simulink model "Allocation_Complex"  (R2015a)
settings: Solver=ode45  StartTime=0.0  StopTime=10.0  RelTol=1e-3
undefined symbols (not defined in the file or in its folder): magnitude
libraries: simulink x16, aerolibutil x10, simulink_extras x6
settings Model: Creator=Nick  LastModifiedBy=Nick

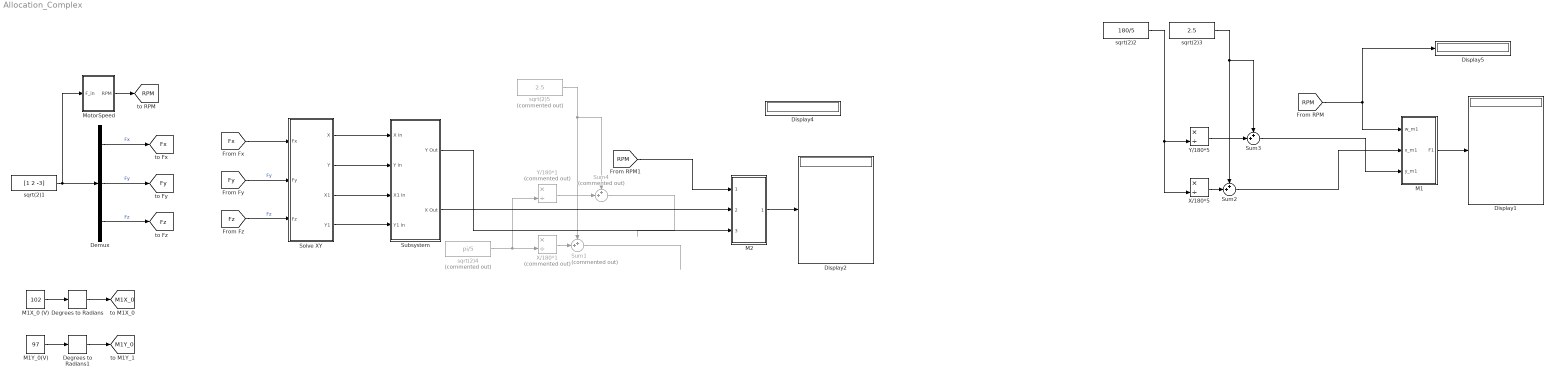
== system Allocation_Complex ==
  Degrees to Radians : simulink_extras/Transformations/Degrees to Radians
  Degrees to Radians1 : simulink_extras/Transformations/Degrees to Radians
  Demux : Demux  Outputs=3
  Display{1..2,4..5} (4 alike) : Display
      settings: Decimation=4
  M1 : Subsystem
  M1X_0 (V) : Constant  Value=102
  M1Y_0(V) : Constant  Value=97
  M2 : Subsystem
  MotorSpeed : Subsystem
  Solve XY : Subsystem
  Subsystem : Subsystem
  Sum1 : Sum  Commented=on  Inputs=++|
  Sum2 : Sum  Inputs=++|
  Sum3 : Sum  Inputs=++|
  Sum4 : Sum  Commented=on  Inputs=++|
  X/180*1 : Product  Commented=on  Inputs=*/
  X/180*5 : Product  Inputs=*/
  Y/180*1 : Product  Commented=on  Inputs=*/
  Y/180*5 : Product  Inputs=*/
  sqrt(2)1 : Constant  Value=[1 2 -3]
  sqrt(2)2 : Constant  Value=180/5
  sqrt(2)3 : Constant  Value=2.5
  sqrt(2)4 : Constant  Commented=on  Value=pi/5
  sqrt(2)5 : Constant  Commented=on  Value=2.5
  tag scope: Fx=global, Fy=global, Fz=global, M1X_0=global, M1Y_0=global, RPM=global
  wires:
  [RPM] -> M1/1(w_m1), Display5/1
  sqrt(2)1/1 -> Demux/1, MotorSpeed/1(F_in)
  sqrt(2)2/1 -> Y/180*5/2, X/180*5/2
  X/180*5/1 -> Sum2/2
  Y/180*5/1 -> Sum3/2
  sqrt(2)3/1 -> Sum3/1, Sum2/1
  M1/1(F1) -> Display1/1
  Sum3/1 -> M1/3(y_m1)
  Sum2/1 -> M1/2(x_m1)
  Demux/1 -> [Fx]  "Fx"
  Demux/2 -> [Fy]  "Fy"
  Demux/3 -> [Fz]  "Fz"
  MotorSpeed/1(RPM) -> [RPM]
  [Fz] -> Solve XY/3(Fz)  "Fz"
  [Fx] -> Solve XY/1(Fx)
  [Fy] -> Solve XY/2(Fy)  "Fy"
  Solve XY/4(Y1) -> Subsystem/4(Y1 in)
  Solve XY/3(X1) -> Subsystem/3(X1 in)
  Solve XY/2(Y) -> Subsystem/2(Y in)
  Solve XY/1(X) -> Subsystem/1(X in)
  M1X_0 (V)/1 -> Degrees to Radians/1
  Degrees to Radians/1 -> [M1X_0]
  M1Y_0(V)/1 -> Degrees to Radians1/1
  Degrees to Radians1/1 -> [M1Y_0]
  [RPM] -> M2/1(w_m1)
  sqrt(2)4/1 -> Y/180*1/2, X/180*1/2
  X/180*1/1 -> Sum1/2
  Y/180*1/1 -> Sum4/2
  sqrt(2)5/1 -> Sum4/1, Sum1/1
  M2/1(Fz_m1) -> Display2/1
  Sum1/1 -> ?
  Sum4/1 -> ?
  Subsystem/1(Y Out) -> M2/3(y_m1)
  Subsystem/2(X Out) -> M2/2(x_m1)

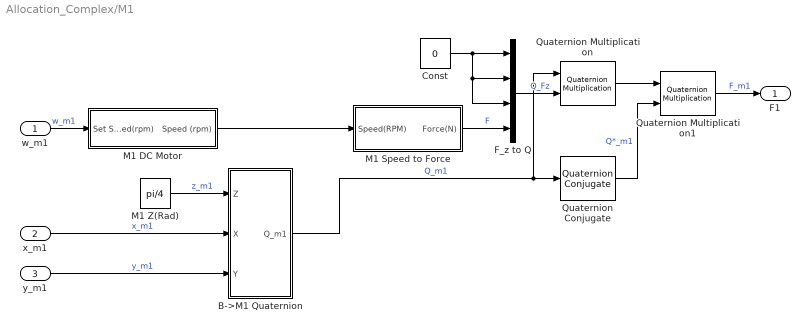
== system Allocation_Complex/M1 ==
  w_m1 : Inport
  x_m1 : Inport  Port=2
  y_m1 : Inport  Port=3
  B->M1 Quaternion : Subsystem
  Const : Constant  Value=0
  F_z to Q : Concatenate  NumInputs=4
  M1 DC Motor : Subsystem
  M1 Speed to Force : Subsystem
  M1 Z(Rad) : Constant  Value=pi/4
  Quaternion Conjugate : aerolibutil/Quaternion Conjugate
  Quaternion Multiplication : aerolibutil/Quaternion Multiplication
  Quaternion Multiplication1 : aerolibutil/Quaternion Multiplication
  F1 : Outport
  wires:
  Quaternion Multiplication/1 -> Quaternion Multiplication1/1
  Const/1 -> F_z to Q/1, F_z to Q/3, F_z to Q/2
  M1 DC Motor/1(Speed (rpm)) -> M1 Speed to Force/1(Speed(RPM))
  B->M1 Quaternion/1(Q_m1) -> Quaternion Conjugate/1, Quaternion Multiplication/1  "Q_m1"
  w_m1/1 -> M1 DC Motor/1(Set Speed(rpm))  "w_m1"
  F_z to Q/1 -> Quaternion Multiplication/2  "Q_Fz"
  M1 Z(Rad)/1 -> B->M1 Quaternion/1("Z ")  "z_m1"
  M1 Speed to Force/1(Force(N)) -> F_z to Q/4  "F"
  y_m1/1 -> B->M1 Quaternion/3(Y)  "y_m1"
  Quaternion Conjugate/1 -> Quaternion Multiplication1/2  "Q*_m1"
  Quaternion Multiplication1/1 -> F1/1  "F_m1"
  x_m1/1 -> B->M1 Quaternion/2(X)  "x_m1"

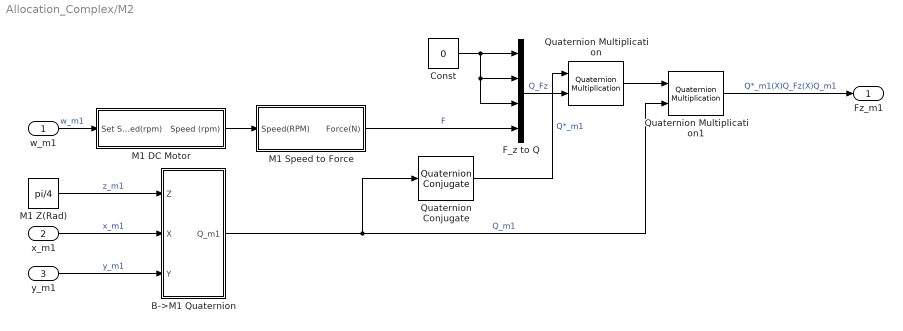
== system Allocation_Complex/M2 ==
  w_m1 : Inport
  x_m1 : Inport  Port=2
  y_m1 : Inport  Port=3
  B->M1 Quaternion : Subsystem
  Const : Constant  Value=0
  F_z to Q : Concatenate  NumInputs=4
  M1 DC Motor : Subsystem
  M1 Speed to Force : Subsystem
  M1 Z(Rad) : Constant  Value=pi/4
  Quaternion Conjugate : aerolibutil/Quaternion Conjugate
  Quaternion Multiplication : aerolibutil/Quaternion Multiplication
  Quaternion Multiplication1 : aerolibutil/Quaternion Multiplication
  Fz_m1 : Outport
  wires:
  Quaternion Multiplication/1 -> Quaternion Multiplication1/1
  Const/1 -> F_z to Q/1, F_z to Q/3, F_z to Q/2
  M1 DC Motor/1(Speed (rpm)) -> M1 Speed to Force/1(Speed(RPM))
  B->M1 Quaternion/1(Q_m1) -> Quaternion Multiplication1/2, Quaternion Conjugate/1  "Q_m1"
  w_m1/1 -> M1 DC Motor/1(Set Speed(rpm))  "w_m1"
  F_z to Q/1 -> Quaternion Multiplication/2  "Q_Fz"
  M1 Z(Rad)/1 -> B->M1 Quaternion/1("Z ")  "z_m1"
  M1 Speed to Force/1(Force(N)) -> F_z to Q/4  "F"
  y_m1/1 -> B->M1 Quaternion/3(Y)  "y_m1"
  Quaternion Multiplication1/1 -> Fz_m1/1  "Q*_m1(X)Q_Fz(X)Q_m1"
  x_m1/1 -> B->M1 Quaternion/2(X)  "x_m1"
  Quaternion Conjugate/1 -> Quaternion Multiplication/1  "Q*_m1"

== system Allocation_Complex/MotorSpeed ==
  F_in : Inport
  Divide : Product  Inputs=*/
  Force Coefficient CT : Constant  Value=0.000243
  Mins : Constant  Value=60
  Product : Product
  w^2 : Sqrt  SaturateOnIntegerOverflow=on
  |F| : Sqrt  SaturateOnIntegerOverflow=on
  |F|^2 : DotProduct  InputSameDT=on  OutDataTypeStr=Inherit: Inherit via internal rule
  RPM : Outport
  wires:
  w^2/1 -> Product/2
  Product/1 -> RPM/1  "RPM"
  Mins/1 -> Product/1
  Divide/1 -> w^2/1
  Force Coefficient CT/1 -> Divide/2
  F_in/1 -> |F|^2/2, |F|^2/1
  |F|^2/1 -> |F|/1
  |F|/1 -> Divide/1

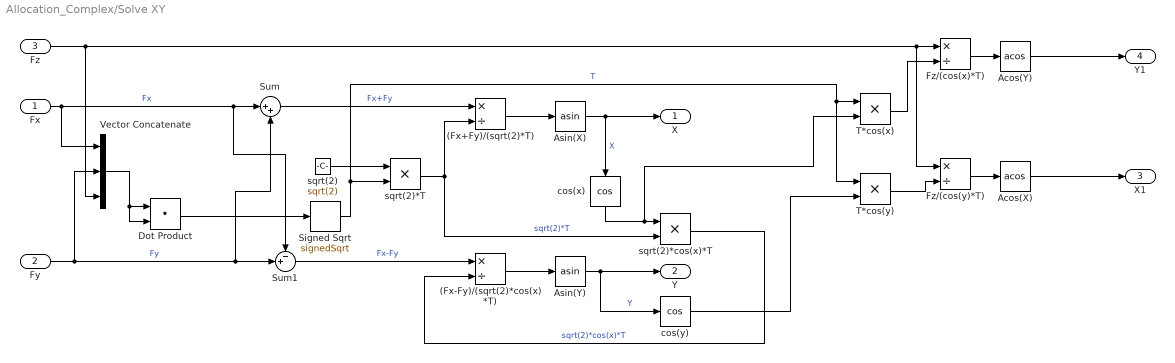
== system Allocation_Complex/Solve XY ==
  Fx : Inport
  Fy : Inport  Port=2
  Fz : Inport  Port=3
  (Fx+Fy)/(sqrt(2)*T) : Product  Inputs=*/
  (Fx-Fy)/(sqrt(2)*cos(x)*T) : Product  Inputs=*/
  Acos(X) : Trigonometry  Operator=acos
  Acos(Y) : Trigonometry  Operator=acos
  Asin(X) : Trigonometry  Operator=asin
  Asin(Y) : Trigonometry  Operator=asin
  Dot Product : DotProduct  InputSameDT=on  OutDataTypeStr=Inherit: Inherit via internal rule
  Fz/(cos(x)*T) : Product  Inputs=*/
  Fz/(cos(y)*T) : Product  Inputs=*/
  Signed Sqrt : Sqrt  Operator=signedSqrt  SaturateOnIntegerOverflow=on
  Sum : Sum  Inputs=|++
  Sum1 : Sum  Inputs=-+|
  T*cos(x) : Product
  T*cos(y) : Product
  Vector Concatenate : Concatenate  NumInputs=3
  cos(x) : Trigonometry  Operator=cos
  cos(y) : Trigonometry  Operator=cos
  sqrt(2) : Constant  Value=sqrt(2)
  sqrt(2)*T : Product
  sqrt(2)*cos(x)*T : Product
  X : Outport
  Y : Outport  Port=2
  X1 : Outport  Port=3
  Y1 : Outport  Port=4
  wires:
  Fy/1 -> Vector Concatenate/2, Sum/2, Sum1/2  "Fy"
  Sum/1 -> (Fx+Fy)/(sqrt(2)*T)/1  "Fx+Fy"
  sqrt(2)/1 -> sqrt(2)*T/1
  T*cos(x)/1 -> Fz/(cos(x)*T)/2
  cos(x)/1 -> sqrt(2)*cos(x)*T/1, T*cos(x)/2
  sqrt(2)*T/1 -> (Fx+Fy)/(sqrt(2)*T)/2, sqrt(2)*cos(x)*T/2  "sqrt(2)*T"
  Fz/(cos(y)*T)/1 -> Acos(X)/1
  (Fx+Fy)/(sqrt(2)*T)/1 -> Asin(X)/1
  cos(y)/1 -> T*cos(y)/2
  sqrt(2)*cos(x)*T/1 -> (Fx-Fy)/(sqrt(2)*cos(x)*T)/2  "sqrt(2)*cos(x)*T"
  (Fx-Fy)/(sqrt(2)*cos(x)*T)/1 -> Asin(Y)/1
  Sum1/1 -> (Fx-Fy)/(sqrt(2)*cos(x)*T)/1  "Fx-Fy"
  Acos(Y)/1 -> Y1/1
  Asin(Y)/1 -> Y/1, cos(y)/1  "Y"
  Fz/(cos(x)*T)/1 -> Acos(Y)/1
  T*cos(y)/1 -> Fz/(cos(y)*T)/2
  Acos(X)/1 -> X1/1
  Asin(X)/1 -> X/1, cos(x)/1  "X"
  Fz/1 -> Vector Concatenate/3, Fz/(cos(y)*T)/1, Fz/(cos(x)*T)/1
  Signed Sqrt/1 -> T*cos(x)/1, T*cos(y)/1, sqrt(2)*T/2  "T"
  Fx/1 -> Sum1/1, Sum/1, Vector Concatenate/1  "Fx"
  Vector Concatenate/1 -> Dot Product/2, Dot Product/1
  Dot Product/1 -> Signed Sqrt/1

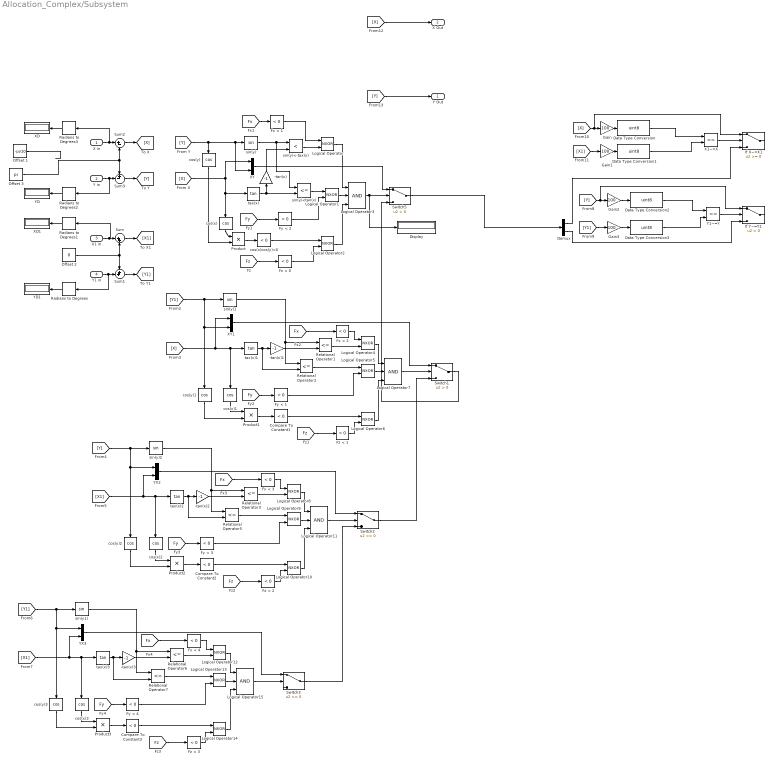
== system Allocation_Complex/Subsystem ==
  X in : Inport
  Y in : Inport  Port=2
  X1 in : Inport  Port=3
  Y1 in : Inport  Port=4
  -tan(x){,1..3} (4 alike) : Gain  Gain=-1
  Compare To Constant1 : simulink/Logic and Bit Operations/Compare To Constant  relop=<  const=0  OutDataTypeStr=boolean
  Compare To Constant2 : simulink/Logic and Bit Operations/Compare To Constant  relop=<  const=0  OutDataTypeStr=boolean
  Compare To Constant3 : simulink/Logic and Bit Operations/Compare To Constant  relop=<  const=0  OutDataTypeStr=boolean
  Data Type Conversion{,1..3} (4 alike) : DataTypeConversion  OutDataTypeStr=uint8
  Demux : Demux  Outputs=2
  Display : Display
  Fx < {1..4} (4 alike) : simulink/Logic and Bit Operations/Compare To Zero  relop=<  OutDataTypeStr=boolean
  Fy < {1..4} (4 alike) : simulink/Logic and Bit Operations/Compare To Zero  relop=<  OutDataTypeStr=boolean
  Fz < {0..3} (4 alike) : simulink/Logic and Bit Operations/Compare To Zero  relop=<  OutDataTypeStr=boolean
  Gain{,1..3} (4 alike) : Gain  Gain=100
  If X~=X1 : Switch
  If Y~=Y1 : Switch  Criteria=u2 > Threshold
  Logical Operator{,1..2,4..6,8..10,12..14} (12 alike) : Logic  Operator=NXOR  AllPortsSameDT=off  OutDataTypeStr=boolean
  Logical Operator{3,7,11,15} (4 alike) : Logic  Inputs=3  AllPortsSameDT=off  OutDataTypeStr=boolean
  Offset 1 : Constant  Value=-pi/10
  Offset 2 : Constant  Value=0
  Offset 3 : Constant  Value=pi
  Product{,1..3} (4 alike) : Product
  Radians to Degrees{,1..3} (4 alike) : simulink_extras/Transformations/Radians to Degrees
  Relational Operator{1..3,5..7} (6 alike) : RelationalOperator  Operator=<=  OutDataTypeStr=boolean
  Sum : Sum  Inputs=|++
  Sum1 : Sum  Inputs=++|
  Sum2 : Sum  Inputs=|+-
  Sum3 : Sum  Inputs=+-|
  Switch1 : Switch  Criteria=u2 > Threshold
  Switch2 : Switch
  Switch3 : Switch
  Switch5 : Switch  Criteria=u2 > Threshold
  X1~=X : RelationalOperator  Operator===  OutDataTypeStr=boolean
  XD : Display
  XD1 : Display
  XY : Concatenate
  XY1 : Concatenate
  Y1~=Y : RelationalOperator  Operator===  OutDataTypeStr=boolean
  YD : Display
  YD1 : Display
  YX2 : Concatenate
  YX3 : Concatenate
  cos(x){,1..3} (4 alike) : Trigonometry  Operator=cos
  cos(x)cos(y)<0 : simulink/Logic and Bit Operations/Compare To Constant  relop=<  const=0  OutDataTypeStr=boolean
  cos(y){,1..3} (4 alike) : Trigonometry  Operator=cos
  sin(y) : Trigonometry
  sin(y)1 : Trigonometry
  sin(y)2 : Trigonometry
  sin(y)<-tax(x) : RelationalOperator  Operator=<  OutDataTypeStr=boolean
  sin(y)<tan(x) : RelationalOperator  Operator=<=  OutDataTypeStr=boolean
  sin(y1) : Trigonometry
  tax(x){,1..3} (4 alike) : Trigonometry  Operator=tan
  Y Out : Outport
  X Out : Outport  Port=2
  wires:
  X1 in/1 -> Radians to Degrees1/1, Sum/1
  Data Type Conversion2/1 -> Y1~=Y/1
  Y1~=Y/1 -> If Y~=Y1/2
  XY/1 -> Switch5/1
  Logical Operator/1 -> Logical Operator3/1
  Logical Operator1/1 -> Logical Operator3/2
  cos(x)cos(y)<0/1 -> Logical Operator2/1
  [X] -> cos(x)/1, tax(x)/1, XY/1
  Product/1 -> cos(x)cos(y)<0/1
  [Y] -> sin(y)/1, XY/2, cos(y)/1
  tax(x)/1 -> sin(y)<tan(x)/2, -tan(x)/1
  cos(y)/1 -> Product/2
  -tan(x)/1 -> sin(y)<-tax(x)/2
  sin(y)/1 -> sin(y)<-tax(x)/1, sin(y)<tan(x)/1
  cos(x)/1 -> Product/1
  [Fy] -> Fy < 2/1
  Fx < 1/1 -> Logical Operator/1
  sin(y)<-tax(x)/1 -> Logical Operator/2
  [Fx] -> Fx < 1/1
  sin(y)<tan(x)/1 -> Logical Operator1/1
  Fy < 2/1 -> Logical Operator1/2
  Logical Operator2/1 -> Logical Operator3/3
  [Fz] -> Fz < 0/1
  Fz < 0/1 -> Logical Operator2/2
  XY1/1 -> Switch1/1
  Logical Operator4/1 -> Logical Operator7/1
  Logical Operator5/1 -> Logical Operator7/2
  Compare To Constant1/1 -> Logical Operator6/1
  [X] -> XY1/1, tax(x)1/1, cos(x)1/1
  Product1/1 -> Compare To Constant1/1
  [Y1] -> sin(y)1/1, cos(y)1/1, XY1/2
  tax(x)1/1 -> -tan(x)1/1, Relational Operator2/2
  cos(y)1/1 -> Product1/2
  -tan(x)1/1 -> Relational Operator1/2
  sin(y)1/1 -> Relational Operator1/1, Relational Operator2/1
  cos(x)1/1 -> Product1/1
  [Fy] -> Fy < 1/1
  Fx < 2/1 -> Logical Operator4/1
  Relational Operator1/1 -> Logical Operator4/2
  [Fx] -> Fx < 2/1
  Relational Operator2/1 -> Logical Operator5/1
  Fy < 1/1 -> Logical Operator5/2
  Logical Operator6/1 -> Logical Operator7/3
  [Fz] -> Fz < 1/1
  Fz < 1/1 -> Logical Operator6/2
  YX2/1 -> Switch2/1
  Logical Operator8/1 -> Logical Operator11/1
  Logical Operator9/1 -> Logical Operator11/2
  Compare To Constant2/1 -> Logical Operator10/1
  [X1] -> tax(x)2/1, cos(x)2/1, YX2/2
  Product2/1 -> Compare To Constant2/1
  tax(x)2/1 -> -tan(x)2/1, Relational Operator5/2
  cos(y)2/1 -> Product2/2
  -tan(x)2/1 -> Relational Operator3/2
  sin(y)2/1 -> Relational Operator3/1, Relational Operator5/1
  cos(x)2/1 -> Product2/1
  [Fy] -> Fy < 3/1
  Fx < 3/1 -> Logical Operator8/1
  Relational Operator3/1 -> Logical Operator8/2
  [Fx] -> Fx < 3/1
  Relational Operator5/1 -> Logical Operator9/1
  Fy < 3/1 -> Logical Operator9/2
  Logical Operator10/1 -> Logical Operator11/3
  [Fz] -> Fz < 2/1
  Fz < 2/1 -> Logical Operator10/2
  YX3/1 -> Switch3/1
  Logical Operator15/1 -> Switch3/2
  Logical Operator12/1 -> Logical Operator15/1
  Logical Operator13/1 -> Logical Operator15/2
  Compare To Constant3/1 -> Logical Operator14/1
  [X1] -> tax(x)3/1, cos(x)3/1, YX3/2
  Product3/1 -> Compare To Constant3/1
  [Y1] -> sin(y1)/1, YX3/1, cos(y)3/1
  tax(x)3/1 -> -tan(x)3/1, Relational Operator7/2
  cos(y)3/1 -> Product3/2
  -tan(x)3/1 -> Relational Operator6/2
  sin(y1)/1 -> Relational Operator6/1, Relational Operator7/1
  cos(x)3/1 -> Product3/1
  [Fy] -> Fy < 4/1
  Fx < 4/1 -> Logical Operator12/1
  Relational Operator6/1 -> Logical Operator12/2
  [Fx] -> Fx < 4/1
  Relational Operator7/1 -> Logical Operator13/1
  Fy < 4/1 -> Logical Operator13/2
  Logical Operator14/1 -> Logical Operator15/3
  [Fz] -> Fz < 3/1
  Fz < 3/1 -> Logical Operator14/2
  [Y] -> sin(y)2/1, YX2/1, cos(y)2/1
  Radians to Degrees/1 -> YD1/1
  Radians to Degrees1/1 -> XD1/1
  Radians to Degrees2/1 -> YD/1
  Radians to Degrees3/1 -> XD/1
  Data Type Conversion1/1 -> X1~=X/2
  X1~=X/1 -> If X~=X1/2
  Switch2/1 -> Switch1/3
  Switch3/1 -> Switch2/3
  Switch5/1 -> Demux/1
  Logical Operator11/1 -> Switch2/2
  Sum/1 -> [X1]
  Sum1/1 -> [Y1]
  Logical Operator3/1 -> Display/1, Switch5/2
  Logical Operator7/1 -> Switch1/2
  Switch1/1 -> Switch5/3
  Data Type Conversion/1 -> X1~=X/1
  Gain/1 -> Data Type Conversion/1
  Gain1/1 -> Data Type Conversion1/1
  [X1] -> Gain1/1
  Gain2/1 -> Data Type Conversion2/1
  Gain3/1 -> Data Type Conversion3/1
  [Y1] -> Gain3/1
  Data Type Conversion3/1 -> Y1~=Y/2
  [X] -> If X~=X1/1, Gain/1
  [Y] -> If Y~=Y1/1, Gain2/1
  Sum2/1 -> [X]
  Sum3/1 -> [Y]
  [Y] -> Y Out/1
  [X] -> X Out/1
  Demux/2 -> If Y~=Y1/3
  Demux/1 -> If X~=X1/3
  X in/1 -> Sum2/1, Radians to Degrees3/1
  Y in/1 -> Radians to Degrees2/1, Sum3/2
  Offset 2/1 -> Sum1/1, Sum/2
  Y1 in/1 -> Radians to Degrees/1, Sum1/2
  Offset 1/1 -> ?
  Offset 3/1 -> Sum2/2, Sum3/1

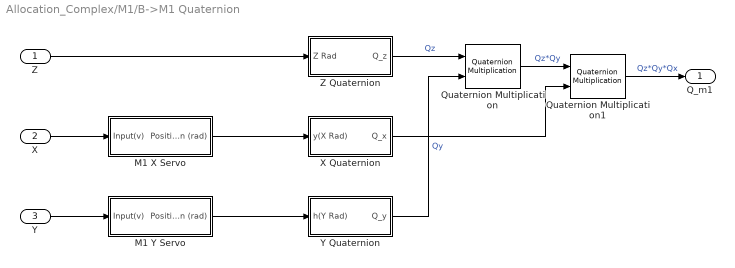
== system Allocation_Complex/M1/B->M1 Quaternion ==
  "Z " : Inport
  X : Inport  Port=2
  Y : Inport  Port=3
  "M1 X Servo " : Subsystem
  M1 Y Servo : Subsystem
  Quaternion Multiplication : aerolibutil/Quaternion Multiplication
  Quaternion Multiplication1 : aerolibutil/Quaternion Multiplication
  X Quaternion : Subsystem
  Y Quaternion : Subsystem
  Z Quaternion : Subsystem
  Q_m1 : Outport
  wires:
  X/1 -> "M1 X Servo "/1(Input(v))
  "M1 X Servo "/1(Position (rad)) -> X Quaternion/1(y(X Rad))
  M1 Y Servo/1(Position (rad)) -> Y Quaternion/1(h(Y Rad))
  "Z "/1 -> Z Quaternion/1(Z Rad)
  Z Quaternion/1(Q_z) -> Quaternion Multiplication/1  "Qz"
  Quaternion Multiplication/1 -> Quaternion Multiplication1/1  "Qz*Qy"
  Quaternion Multiplication1/1 -> Q_m1/1  "Qz*Qy*Qx"
  Y/1 -> M1 Y Servo/1(Input(v))
  Y Quaternion/1(Q_y) -> Quaternion Multiplication/2  "Qy"
  X Quaternion/1(Q_x) -> Quaternion Multiplication1/2

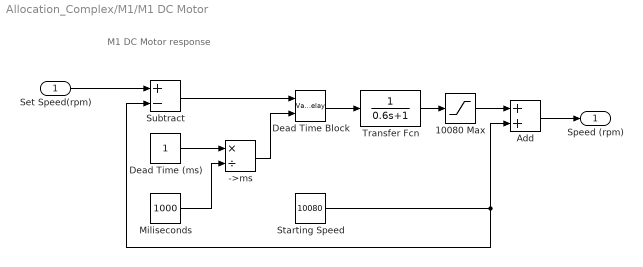
== system Allocation_Complex/M1/M1 DC Motor ==
  note: M1 DC Motor response
  Set Speed(rpm) : Inport
  ->ms : Product  Inputs=*/
  10080 Max : Saturate  UpperLimit=10080  LowerLimit=-10080
  Add : Sum
  Dead Time (ms) : Constant
  Dead Time Block : VariableTransportDelay  MaximumDelay=10
  Miliseconds : Constant  Value=1000
  Starting Speed : Constant  Value=10080
  Subtract : Sum  Inputs=+-
  Transfer Fcn : TransferFcn  Numerator=1  Denominator=[0.6 1]
  Speed (rpm) : Outport
  wires:
  Dead Time Block/1 -> Transfer Fcn/1
  Miliseconds/1 -> ->ms/2
  Dead Time (ms)/1 -> ->ms/1
  ->ms/1 -> Dead Time Block/2
  Transfer Fcn/1 -> 10080 Max/1
  Set Speed(rpm)/1 -> Subtract/1
  10080 Max/1 -> Add/1
  Add/1 -> Speed (rpm)/1
  Starting Speed/1 -> Subtract/2, Add/2
  Subtract/1 -> Dead Time Block/1

== system Allocation_Complex/M1/M1 Speed to Force ==
  note: RPS to Force
  Speed(RPM) : Inport
  ->RPS : Product  Inputs=*/
  Force Coefficient CT : Constant  Value=0.000243
  M1 w^2 : Math  Operator=magnitude^2  SaturateOnIntegerOverflow=on
  Mins : Constant  Value=60
  Product : Product
  Force(N) : Outport
  wires:
  M1 w^2/1 -> Product/2
  ->RPS/1 -> M1 w^2/1
  Speed(RPM)/1 -> ->RPS/1
  Force Coefficient CT/1 -> Product/1
  Mins/1 -> ->RPS/2
  Product/1 -> Force(N)/1

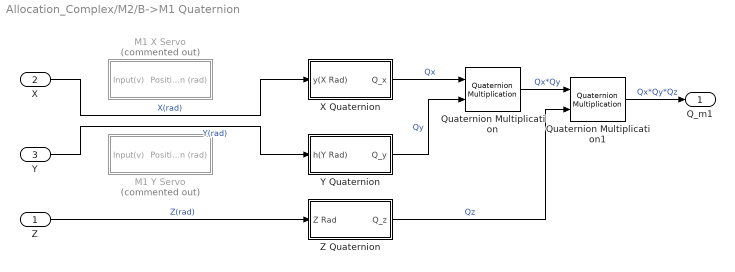
== system Allocation_Complex/M2/B->M1 Quaternion ==
  "Z " : Inport
  X : Inport  Port=2
  Y : Inport  Port=3
  "M1 X Servo " : Subsystem  Commented=on
  M1 Y Servo : Subsystem  Commented=on
  Quaternion Multiplication : aerolibutil/Quaternion Multiplication
  Quaternion Multiplication1 : aerolibutil/Quaternion Multiplication
  X Quaternion : Subsystem
  Y Quaternion : Subsystem
  Z Quaternion : Subsystem
  Q_m1 : Outport
  wires:
  X/1 -> X Quaternion/1(y(X Rad))  "X(rad)"
  "Z "/1 -> Z Quaternion/1(Z Rad)  "Z(rad)"
  Quaternion Multiplication/1 -> Quaternion Multiplication1/1  "Qx*Qy"
  Quaternion Multiplication1/1 -> Q_m1/1  "Qx*Qy*Qz"
  Y/1 -> Y Quaternion/1(h(Y Rad))  "Y(rad)"
  X Quaternion/1(Q_x) -> Quaternion Multiplication/1  "Qx"
  Y Quaternion/1(Q_y) -> Quaternion Multiplication/2  "Qy"
  Z Quaternion/1(Q_z) -> Quaternion Multiplication1/2  "Qz"

== system Allocation_Complex/M2/M1 DC Motor ==
  note: M1 DC Motor response
  Set Speed(rpm) : Inport
  ->ms : Product  Inputs=*/
  10080 Max : Saturate  UpperLimit=10080  LowerLimit=-10080
  Add : Sum
  Dead Time (ms) : Constant
  Dead Time Block : VariableTransportDelay  MaximumDelay=10
  Miliseconds : Constant  Value=1000
  Starting Speed : Constant  Value=10080
  Subtract : Sum  Inputs=+-
  Transfer Fcn : TransferFcn  Numerator=1  Denominator=[0.6 1]
  Speed (rpm) : Outport
  wires:
  Dead Time Block/1 -> Transfer Fcn/1
  Miliseconds/1 -> ->ms/2
  Dead Time (ms)/1 -> ->ms/1
  ->ms/1 -> Dead Time Block/2
  Transfer Fcn/1 -> 10080 Max/1
  Set Speed(rpm)/1 -> Subtract/1
  10080 Max/1 -> Add/1
  Add/1 -> Speed (rpm)/1
  Starting Speed/1 -> Add/2, Subtract/2
  Subtract/1 -> Dead Time Block/1

== system Allocation_Complex/M2/M1 Speed to Force ==
  note: RPS to Force
  Speed(RPM) : Inport
  ->RPS : Product  Inputs=*/
  Force Coefficient CT : Constant  Value=0.000243
  M1 w^2 : Math  Operator=magnitude^2  SaturateOnIntegerOverflow=on
  Mins : Constant  Value=60
  Product : Product
  Force(N) : Outport
  wires:
  M1 w^2/1 -> Product/2
  ->RPS/1 -> M1 w^2/1
  Speed(RPM)/1 -> ->RPS/1
  Force Coefficient CT/1 -> Product/1
  Mins/1 -> ->RPS/2
  Product/1 -> Force(N)/1

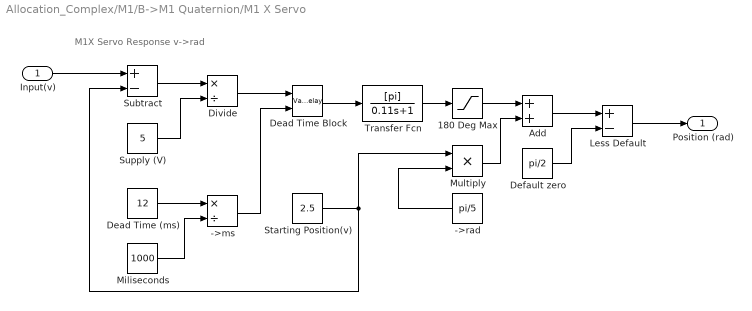
== system Allocation_Complex/M1/B->M1 Quaternion/M1 X Servo  ==
  note: M1X Servo Response v->rad
  Input(v) : Inport
  ->ms : Product  Inputs=*/
  ->rad : Constant  Value=pi/5
  180 Deg Max : Saturate  UpperLimit=pi/2  LowerLimit=-pi/2
  Add : Sum
  Dead Time (ms) : Constant  Value=12
  Dead Time Block : VariableTransportDelay  MaximumDelay=10
  Default zero : Constant  Value=pi/2
  Divide : Product  Inputs=*/
  Less Default : Sum  Inputs=+-
  Miliseconds : Constant  Value=1000
  Multiply : Product  Inputs=**
  Starting Position(v) : Constant  Value=2.5
  Subtract : Sum  Inputs=+-
  Supply (V) : Constant  Value=5
  Transfer Fcn : TransferFcn  Numerator=[pi]  Denominator=[0.11 1]
  Position (rad) : Outport
  wires:
  Miliseconds/1 -> ->ms/2
  Dead Time (ms)/1 -> ->ms/1
  Default zero/1 -> Less Default/2
  Starting Position(v)/1 -> Multiply/1, Subtract/2
  Subtract/1 -> Divide/1
  Supply (V)/1 -> Divide/2
  Divide/1 -> Dead Time Block/1
  ->ms/1 -> Dead Time Block/2
  Dead Time Block/1 -> Transfer Fcn/1
  Transfer Fcn/1 -> 180 Deg Max/1
  180 Deg Max/1 -> Add/1
  ->rad/1 -> Multiply/2
  Multiply/1 -> Add/2
  Less Default/1 -> Position (rad)/1
  Add/1 -> Less Default/1
  Input(v)/1 -> Subtract/1

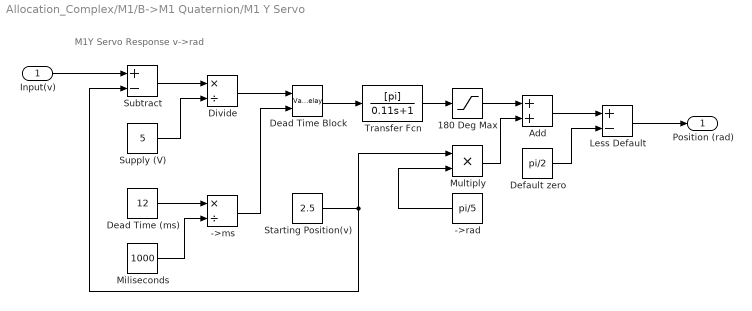
== system Allocation_Complex/M1/B->M1 Quaternion/M1 Y Servo ==
  note: M1Y Servo Response v->rad
  Input(v) : Inport
  ->ms : Product  Inputs=*/
  ->rad : Constant  Value=pi/5
  180 Deg Max : Saturate  UpperLimit=pi/2  LowerLimit=-pi/2
  Add : Sum
  Dead Time (ms) : Constant  Value=12
  Dead Time Block : VariableTransportDelay  MaximumDelay=10
  Default zero : Constant  Value=pi/2
  Divide : Product  Inputs=*/
  Less Default : Sum  Inputs=+-
  Miliseconds : Constant  Value=1000
  Multiply : Product  Inputs=**
  Starting Position(v) : Constant  Value=2.5
  Subtract : Sum  Inputs=+-
  Supply (V) : Constant  Value=5
  Transfer Fcn : TransferFcn  Numerator=[pi]  Denominator=[0.11 1]
  Position (rad) : Outport
  wires:
  Miliseconds/1 -> ->ms/2
  Dead Time (ms)/1 -> ->ms/1
  Default zero/1 -> Less Default/2
  Starting Position(v)/1 -> Multiply/1, Subtract/2
  Subtract/1 -> Divide/1
  Supply (V)/1 -> Divide/2
  Divide/1 -> Dead Time Block/1
  ->ms/1 -> Dead Time Block/2
  Dead Time Block/1 -> Transfer Fcn/1
  Transfer Fcn/1 -> 180 Deg Max/1
  180 Deg Max/1 -> Add/1
  ->rad/1 -> Multiply/2
  Multiply/1 -> Add/2
  Less Default/1 -> Position (rad)/1
  Add/1 -> Less Default/1
  Input(v)/1 -> Subtract/1

== system Allocation_Complex/M1/B->M1 Quaternion/X Quaternion ==
  y(X Rad) : Inport
  Const : Constant  Value=2
  Const1 : Constant  Value=0
  Divide : Product  Inputs=*/
  Trigonometric Function : Trigonometry  Operator=cos
  Trigonometric Function1 : Trigonometry
  Vector Concatenate : Concatenate  NumInputs=4
  Q_x : Outport
  wires:
  Vector Concatenate/1 -> Q_x/1
  Const/1 -> Divide/2
  Trigonometric Function1/1 -> Vector Concatenate/2
  Trigonometric Function/1 -> Vector Concatenate/1
  Const1/1 -> Vector Concatenate/4, Vector Concatenate/3
  Divide/1 -> Trigonometric Function1/1, Trigonometric Function/1
  y(X Rad)/1 -> Divide/1

== system Allocation_Complex/M1/B->M1 Quaternion/Y Quaternion ==
  h(Y Rad) : Inport
  Const : Constant  Value=2
  Const1 : Constant  Value=0
  Divide : Product  Inputs=*/
  Trigonometric Function : Trigonometry  Operator=cos
  Trigonometric Function1 : Trigonometry
  Vector Concatenate : Concatenate  NumInputs=4
  Q_y : Outport
  wires:
  Vector Concatenate/1 -> Q_y/1
  Const/1 -> Divide/2
  Trigonometric Function/1 -> Vector Concatenate/1
  Const1/1 -> Vector Concatenate/2, Vector Concatenate/4
  Divide/1 -> Trigonometric Function1/1, Trigonometric Function/1
  h(Y Rad)/1 -> Divide/1
  Trigonometric Function1/1 -> Vector Concatenate/3

== system Allocation_Complex/M1/B->M1 Quaternion/Z Quaternion ==
  Z Rad : Inport
  Const : Constant  Value=2
  Const1 : Constant  Value=0
  Divide : Product  Inputs=*/
  Trigonometric Function : Trigonometry  Operator=cos
  Trigonometric Function1 : Trigonometry
  Vector Concatenate : Concatenate  NumInputs=4
  Q_z : Outport
  wires:
  Vector Concatenate/1 -> Q_z/1
  Const/1 -> Divide/2
  Trigonometric Function/1 -> Vector Concatenate/1
  Const1/1 -> Vector Concatenate/3, Vector Concatenate/2
  Divide/1 -> Trigonometric Function1/1, Trigonometric Function/1
  Z Rad/1 -> Divide/1
  Trigonometric Function1/1 -> Vector Concatenate/4

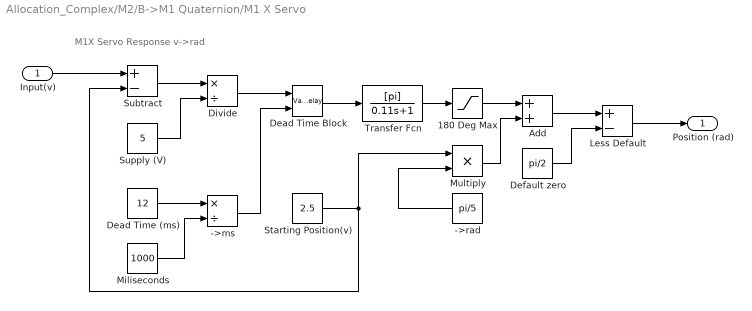
== system Allocation_Complex/M2/B->M1 Quaternion/M1 X Servo  ==
  note: M1X Servo Response v->rad
  Input(v) : Inport
  ->ms : Product  Inputs=*/
  ->rad : Constant  Value=pi/5
  180 Deg Max : Saturate  UpperLimit=pi  LowerLimit=-pi
  Add : Sum
  Dead Time (ms) : Constant  Value=12
  Dead Time Block : VariableTransportDelay  MaximumDelay=10
  Default zero : Constant  Value=pi/2
  Divide : Product  Inputs=*/
  Less Default : Sum  Inputs=+-
  Miliseconds : Constant  Value=1000
  Multiply : Product  Inputs=**
  Starting Position(v) : Constant  Value=2.5
  Subtract : Sum  Inputs=+-
  Supply (V) : Constant  Value=5
  Transfer Fcn : TransferFcn  Numerator=[pi]  Denominator=[0.11 1]
  Position (rad) : Outport
  wires:
  Miliseconds/1 -> ->ms/2
  Dead Time (ms)/1 -> ->ms/1
  Default zero/1 -> Less Default/2
  Starting Position(v)/1 -> Multiply/1, Subtract/2
  Subtract/1 -> Divide/1
  Supply (V)/1 -> Divide/2
  Divide/1 -> Dead Time Block/1
  ->ms/1 -> Dead Time Block/2
  Dead Time Block/1 -> Transfer Fcn/1
  Transfer Fcn/1 -> 180 Deg Max/1
  180 Deg Max/1 -> Add/1
  ->rad/1 -> Multiply/2
  Multiply/1 -> Add/2
  Less Default/1 -> Position (rad)/1
  Add/1 -> Less Default/1
  Input(v)/1 -> Subtract/1

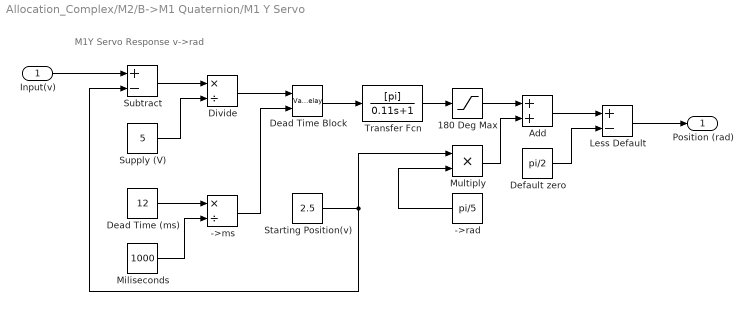
== system Allocation_Complex/M2/B->M1 Quaternion/M1 Y Servo ==
  note: M1Y Servo Response v->rad
  Input(v) : Inport
  ->ms : Product  Inputs=*/
  ->rad : Constant  Value=pi/5
  180 Deg Max : Saturate  UpperLimit=pi  LowerLimit=-pi
  Add : Sum
  Dead Time (ms) : Constant  Value=12
  Dead Time Block : VariableTransportDelay  MaximumDelay=10
  Default zero : Constant  Value=pi/2
  Divide : Product  Inputs=*/
  Less Default : Sum  Inputs=+-
  Miliseconds : Constant  Value=1000
  Multiply : Product  Inputs=**
  Starting Position(v) : Constant  Value=2.5
  Subtract : Sum  Inputs=+-
  Supply (V) : Constant  Value=5
  Transfer Fcn : TransferFcn  Numerator=[pi]  Denominator=[0.11 1]
  Position (rad) : Outport
  wires:
  Miliseconds/1 -> ->ms/2
  Dead Time (ms)/1 -> ->ms/1
  Default zero/1 -> Less Default/2
  Starting Position(v)/1 -> Multiply/1, Subtract/2
  Subtract/1 -> Divide/1
  Supply (V)/1 -> Divide/2
  Divide/1 -> Dead Time Block/1
  ->ms/1 -> Dead Time Block/2
  Dead Time Block/1 -> Transfer Fcn/1
  Transfer Fcn/1 -> 180 Deg Max/1
  180 Deg Max/1 -> Add/1
  ->rad/1 -> Multiply/2
  Multiply/1 -> Add/2
  Less Default/1 -> Position (rad)/1
  Add/1 -> Less Default/1
  Input(v)/1 -> Subtract/1

== system Allocation_Complex/M2/B->M1 Quaternion/X Quaternion ==
  y(X Rad) : Inport
  Const : Constant  Value=2
  Const1 : Constant  Value=0
  Divide : Product  Inputs=*/
  Trigonometric Function : Trigonometry  Operator=cos
  Trigonometric Function1 : Trigonometry
  Vector Concatenate : Concatenate  NumInputs=4
  Q_x : Outport
  wires:
  Vector Concatenate/1 -> Q_x/1
  Const/1 -> Divide/2
  Trigonometric Function1/1 -> Vector Concatenate/2
  Trigonometric Function/1 -> Vector Concatenate/1
  Const1/1 -> Vector Concatenate/4, Vector Concatenate/3
  Divide/1 -> Trigonometric Function1/1, Trigonometric Function/1
  y(X Rad)/1 -> Divide/1

== system Allocation_Complex/M2/B->M1 Quaternion/Y Quaternion ==
  h(Y Rad) : Inport
  Const : Constant  Value=2
  Const1 : Constant  Value=0
  Divide : Product  Inputs=*/
  Trigonometric Function : Trigonometry  Operator=cos
  Trigonometric Function1 : Trigonometry
  Vector Concatenate : Concatenate  NumInputs=4
  Q_y : Outport
  wires:
  Vector Concatenate/1 -> Q_y/1
  Const/1 -> Divide/2
  Trigonometric Function/1 -> Vector Concatenate/1
  Const1/1 -> Vector Concatenate/2, Vector Concatenate/4
  Divide/1 -> Trigonometric Function1/1, Trigonometric Function/1
  h(Y Rad)/1 -> Divide/1
  Trigonometric Function1/1 -> Vector Concatenate/3

== system Allocation_Complex/M2/B->M1 Quaternion/Z Quaternion ==
  Z Rad : Inport
  Const : Constant  Value=2
  Const1 : Constant  Value=0
  Divide : Product  Inputs=*/
  Trigonometric Function : Trigonometry  Operator=cos
  Trigonometric Function1 : Trigonometry
  Vector Concatenate : Concatenate  NumInputs=4
  Q_z : Outport
  wires:
  Vector Concatenate/1 -> Q_z/1
  Const/1 -> Divide/2
  Trigonometric Function/1 -> Vector Concatenate/1
  Const1/1 -> Vector Concatenate/3, Vector Concatenate/2
  Divide/1 -> Trigonometric Function1/1, Trigonometric Function/1
  Z Rad/1 -> Divide/1
  Trigonometric Function1/1 -> Vector Concatenate/4
